simulink model "A_2_7_TFBasedSimulationslx"  (R2024b)
settings: Solver=VariableStepAuto  StartTime=0.0  StopTime=10.0  RelTol=1e-3
values from neighbouring files (symbols this model uses):
  aileronStep = deg2rad(0.8)    [A_2_7_TFBasedSimulation.m]
  ruderStep = deg2rad(1.2)    [A_2_7_TFBasedSimulation.m]
libraries: cstblocks x2
settings Model: Creator=the_main  LastModifiedBy=the_main

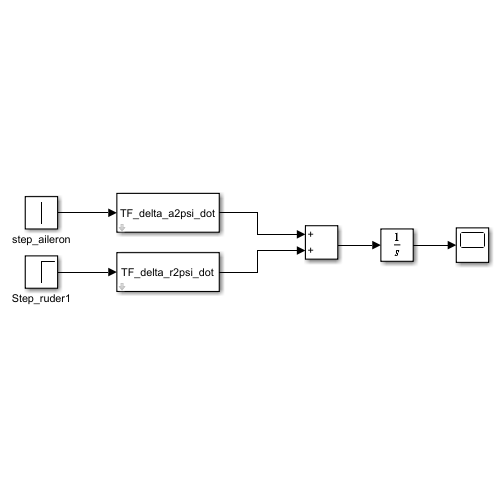
[thumbnail: Simulink's stored preview of the top-level diagram]
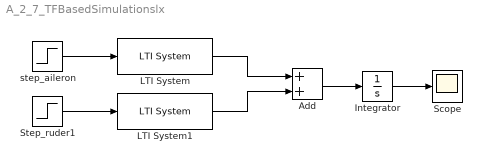
== system A_2_7_TFBasedSimulationslx ==
  Add : Sum
  Integrator : Integrator
  LTI System : cstblocks/LTI System  sys=TF_delta_a2psi_dot  IC=[]  PadeOrder=0
  LTI System1 : cstblocks/LTI System  sys=TF_delta_r2psi_dot  IC=[]  PadeOrder=0
  Scope : Scope
  Step_ruder1 : Step  After=ruderStep  SampleTime=0
  step_aileron : Step  After=aileronStep  SampleTime=0
  wires:
  LTI System/1 -> Add/1
  LTI System1/1 -> Add/2
  Add/1 -> Integrator/1
  Integrator/1 -> Scope/1
  step_aileron/1 -> LTI System/1
  Step_ruder1/1 -> LTI System1/1
